simulink model "test_final_sift"  (R2015a)
settings: Solver=ode45  StartTime=0.0  StopTime=10.0  RelTol=1e-3
InitFcn:
  | %% DSPBuilder Start
  | alt_dspbuilder_update_model(bdroot)
  | %% DSPBuilder End
libraries: allblocks_alteradspbuilder2 x2309
(part 13 of 27)

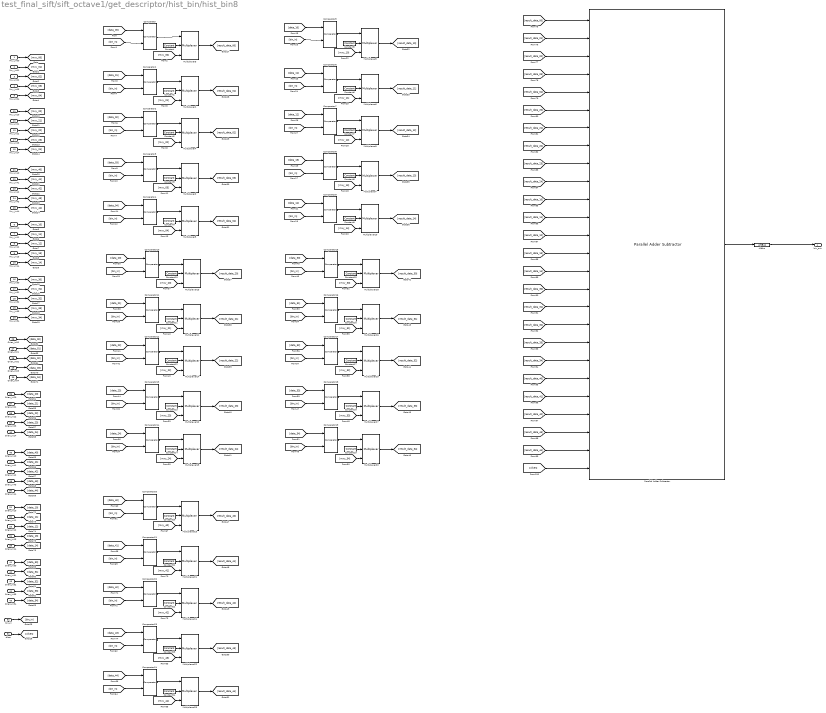
== system test_final_sift/sift_octave1/get_descriptor/hist_bin/hist_bin8 ==
  Mxy_In00 : Inport
  Mxy_In01 : Inport  Port=2
  Mxy_In02 : Inport  Port=3
  Mxy_In03 : Inport  Port=4
  Mxy_In04 : Inport  Port=5
  Mxy_In10 : Inport  Port=6
  Mxy_In11 : Inport  Port=7
  Mxy_In12 : Inport  Port=8
  Mxy_In13 : Inport  Port=9
  Mxy_In14 : Inport  Port=10
  Mxy_In20 : Inport  Port=11
  Mxy_In21 : Inport  Port=12
  Mxy_In22 : Inport  Port=13
  Mxy_In23 : Inport  Port=14
  Mxy_In24 : Inport  Port=15
  Mxy_In30 : Inport  Port=16
  Mxy_In31 : Inport  Port=17
  Mxy_In32 : Inport  Port=18
  Mxy_In33 : Inport  Port=19
  Mxy_In34 : Inport  Port=20
  Mxy_In40 : Inport  Port=21
  Mxy_In41 : Inport  Port=22
  Mxy_In42 : Inport  Port=23
  Mxy_In43 : Inport  Port=24
  Mxy_In44 : Inport  Port=25
  Orien_In00 : Inport  Port=26
  Orien_In01 : Inport  Port=27
  Orien_In02 : Inport  Port=28
  Orien_In03 : Inport  Port=29
  Orien_In04 : Inport  Port=30
  Orien_In10 : Inport  Port=31
  Orien_In11 : Inport  Port=32
  Orien_In12 : Inport  Port=33
  Orien_In13 : Inport  Port=34
  Orien_In14 : Inport  Port=35
  Orien_In20 : Inport  Port=36
  Orien_In21 : Inport  Port=37
  Orien_In22 : Inport  Port=38
  Orien_In23 : Inport  Port=39
  Orien_In24 : Inport  Port=40
  Orien_In30 : Inport  Port=41
  Orien_In31 : Inport  Port=42
  Orien_In32 : Inport  Port=43
  Orien_In33 : Inport  Port=44
  Orien_In34 : Inport  Port=45
  Orien_In40 : Inport  Port=46
  Orien_In41 : Inport  Port=47
  Orien_In42 : Inport  Port=48
  Orien_In43 : Inport  Port=49
  Orien_In44 : Inport  Port=50
  clken : Inport  Port=51
  bin_in : Inport  Port=52
  AltBus : allblocks_alteradspbuilder2/AltBus  BusType=Unsigned Integer  bwl=16  bwr=0  saturate=off  floatingPointInput=on  floatingPointOutput=on  logOutputs=off  logFile=C:\Users\ASUS\Desktop\sift_fpga\Octave_2\tb_test_final_sift\test%5Ffinal%5Fsift_sift%5Foctave1_get%5Fdescriptor_hist%5Fbin_hist%5Fbin8_AltBus.fixedpointlog
  Comparator : allblocks_alteradspbuilder2/Comparator  direction=a == b  pipeline_display=0  allowFloatingPointOverride=on  logOutputs=off  logFile=C:\Users\ASUS\Desktop\sift_fpga\Octave_2\tb_test_final_sift\test%5Ffinal%5Fsift_sift%5Foctave1_get%5Fdescriptor_hist%5Fbin_hist%5Fbin8_Comparator.fixedpointlog
  Comparator1 : allblocks_alteradspbuilder2/Comparator  direction=a == b  pipeline_display=0  allowFloatingPointOverride=on  logOutputs=off  logFile=C:\Users\ASUS\Desktop\sift_fpga\Octave_2\tb_test_final_sift\test%5Ffinal%5Fsift_sift%5Foctave1_get%5Fdescriptor_hist%5Fbin_hist%5Fbin8_Comparator1.fixedpointlog
  Comparator10 : allblocks_alteradspbuilder2/Comparator  direction=a == b  pipeline_display=0  allowFloatingPointOverride=on  logOutputs=off  logFile=C:\Users\ASUS\Desktop\sift_fpga\Octave_2\tb_test_final_sift\test%5Ffinal%5Fsift_sift%5Foctave1_get%5Fdescriptor_hist%5Fbin_hist%5Fbin8_Comparator10.fixedpointlog
  Comparator11 : allblocks_alteradspbuilder2/Comparator  direction=a == b  pipeline_display=0  allowFloatingPointOverride=on  logOutputs=off  logFile=C:\Users\ASUS\Desktop\sift_fpga\Octave_2\tb_test_final_sift\test%5Ffinal%5Fsift_sift%5Foctave1_get%5Fdescriptor_hist%5Fbin_hist%5Fbin8_Comparator11.fixedpointlog
  Comparator12 : allblocks_alteradspbuilder2/Comparator  direction=a == b  pipeline_display=0  allowFloatingPointOverride=on  logOutputs=off  logFile=C:\Users\ASUS\Desktop\sift_fpga\Octave_2\tb_test_final_sift\test%5Ffinal%5Fsift_sift%5Foctave1_get%5Fdescriptor_hist%5Fbin_hist%5Fbin8_Comparator12.fixedpointlog
  Comparator13 : allblocks_alteradspbuilder2/Comparator  direction=a == b  pipeline_display=0  allowFloatingPointOverride=on  logOutputs=off  logFile=C:\Users\ASUS\Desktop\sift_fpga\Octave_2\tb_test_final_sift\test%5Ffinal%5Fsift_sift%5Foctave1_get%5Fdescriptor_hist%5Fbin_hist%5Fbin8_Comparator13.fixedpointlog
  Comparator14 : allblocks_alteradspbuilder2/Comparator  direction=a == b  pipeline_display=0  allowFloatingPointOverride=on  logOutputs=off  logFile=C:\Users\ASUS\Desktop\sift_fpga\Octave_2\tb_test_final_sift\test%5Ffinal%5Fsift_sift%5Foctave1_get%5Fdescriptor_hist%5Fbin_hist%5Fbin8_Comparator14.fixedpointlog
  Comparator15 : allblocks_alteradspbuilder2/Comparator  direction=a == b  pipeline_display=0  allowFloatingPointOverride=on  logOutputs=off  logFile=C:\Users\ASUS\Desktop\sift_fpga\Octave_2\tb_test_final_sift\test%5Ffinal%5Fsift_sift%5Foctave1_get%5Fdescriptor_hist%5Fbin_hist%5Fbin8_Comparator15.fixedpointlog
  Comparator16 : allblocks_alteradspbuilder2/Comparator  direction=a == b  pipeline_display=0  allowFloatingPointOverride=on  logOutputs=off  logFile=C:\Users\ASUS\Desktop\sift_fpga\Octave_2\tb_test_final_sift\test%5Ffinal%5Fsift_sift%5Foctave1_get%5Fdescriptor_hist%5Fbin_hist%5Fbin8_Comparator16.fixedpointlog
  Comparator17 : allblocks_alteradspbuilder2/Comparator  direction=a == b  pipeline_display=0  allowFloatingPointOverride=on  logOutputs=off  logFile=C:\Users\ASUS\Desktop\sift_fpga\Octave_2\tb_test_final_sift\test%5Ffinal%5Fsift_sift%5Foctave1_get%5Fdescriptor_hist%5Fbin_hist%5Fbin8_Comparator17.fixedpointlog
  Comparator18 : allblocks_alteradspbuilder2/Comparator  direction=a == b  pipeline_display=0  allowFloatingPointOverride=on  logOutputs=off  logFile=C:\Users\ASUS\Desktop\sift_fpga\Octave_2\tb_test_final_sift\test%5Ffinal%5Fsift_sift%5Foctave1_get%5Fdescriptor_hist%5Fbin_hist%5Fbin8_Comparator18.fixedpointlog
  Comparator19 : allblocks_alteradspbuilder2/Comparator  direction=a == b  pipeline_display=0  allowFloatingPointOverride=on  logOutputs=off  logFile=C:\Users\ASUS\Desktop\sift_fpga\Octave_2\tb_test_final_sift\test%5Ffinal%5Fsift_sift%5Foctave1_get%5Fdescriptor_hist%5Fbin_hist%5Fbin8_Comparator19.fixedpointlog
  Comparator2 : allblocks_alteradspbuilder2/Comparator  direction=a == b  pipeline_display=0  allowFloatingPointOverride=on  logOutputs=off  logFile=C:\Users\ASUS\Desktop\sift_fpga\Octave_2\tb_test_final_sift\test%5Ffinal%5Fsift_sift%5Foctave1_get%5Fdescriptor_hist%5Fbin_hist%5Fbin8_Comparator2.fixedpointlog
  Comparator20 : allblocks_alteradspbuilder2/Comparator  direction=a == b  pipeline_display=0  allowFloatingPointOverride=on  logOutputs=off  logFile=C:\Users\ASUS\Desktop\sift_fpga\Octave_2\tb_test_final_sift\test%5Ffinal%5Fsift_sift%5Foctave1_get%5Fdescriptor_hist%5Fbin_hist%5Fbin8_Comparator20.fixedpointlog
  Comparator21 : allblocks_alteradspbuilder2/Comparator  direction=a == b  pipeline_display=0  allowFloatingPointOverride=on  logOutputs=off  logFile=C:\Users\ASUS\Desktop\sift_fpga\Octave_2\tb_test_final_sift\test%5Ffinal%5Fsift_sift%5Foctave1_get%5Fdescriptor_hist%5Fbin_hist%5Fbin8_Comparator21.fixedpointlog
  Comparator22 : allblocks_alteradspbuilder2/Comparator  direction=a == b  pipeline_display=0  allowFloatingPointOverride=on  logOutputs=off  logFile=C:\Users\ASUS\Desktop\sift_fpga\Octave_2\tb_test_final_sift\test%5Ffinal%5Fsift_sift%5Foctave1_get%5Fdescriptor_hist%5Fbin_hist%5Fbin8_Comparator22.fixedpointlog
  Comparator23 : allblocks_alteradspbuilder2/Comparator  direction=a == b  pipeline_display=0  allowFloatingPointOverride=on  logOutputs=off  logFile=C:\Users\ASUS\Desktop\sift_fpga\Octave_2\tb_test_final_sift\test%5Ffinal%5Fsift_sift%5Foctave1_get%5Fdescriptor_hist%5Fbin_hist%5Fbin8_Comparator23.fixedpointlog
  Comparator24 : allblocks_alteradspbuilder2/Comparator  direction=a == b  pipeline_display=0  allowFloatingPointOverride=on  logOutputs=off  logFile=C:\Users\ASUS\Desktop\sift_fpga\Octave_2\tb_test_final_sift\test%5Ffinal%5Fsift_sift%5Foctave1_get%5Fdescriptor_hist%5Fbin_hist%5Fbin8_Comparator24.fixedpointlog
  Comparator3 : allblocks_alteradspbuilder2/Comparator  direction=a == b  pipeline_display=0  allowFloatingPointOverride=on  logOutputs=off  logFile=C:\Users\ASUS\Desktop\sift_fpga\Octave_2\tb_test_final_sift\test%5Ffinal%5Fsift_sift%5Foctave1_get%5Fdescriptor_hist%5Fbin_hist%5Fbin8_Comparator3.fixedpointlog
  Comparator4 : allblocks_alteradspbuilder2/Comparator  direction=a == b  pipeline_display=0  allowFloatingPointOverride=on  logOutputs=off  logFile=C:\Users\ASUS\Desktop\sift_fpga\Octave_2\tb_test_final_sift\test%5Ffinal%5Fsift_sift%5Foctave1_get%5Fdescriptor_hist%5Fbin_hist%5Fbin8_Comparator4.fixedpointlog
  Comparator5 : allblocks_alteradspbuilder2/Comparator  direction=a == b  pipeline_display=0  allowFloatingPointOverride=on  logOutputs=off  logFile=C:\Users\ASUS\Desktop\sift_fpga\Octave_2\tb_test_final_sift\test%5Ffinal%5Fsift_sift%5Foctave1_get%5Fdescriptor_hist%5Fbin_hist%5Fbin8_Comparator5.fixedpointlog
  Comparator6 : allblocks_alteradspbuilder2/Comparator  direction=a == b  pipeline_display=0  allowFloatingPointOverride=on  logOutputs=off  logFile=C:\Users\ASUS\Desktop\sift_fpga\Octave_2\tb_test_final_sift\test%5Ffinal%5Fsift_sift%5Foctave1_get%5Fdescriptor_hist%5Fbin_hist%5Fbin8_Comparator6.fixedpointlog
  Comparator7 : allblocks_alteradspbuilder2/Comparator  direction=a == b  pipeline_display=0  allowFloatingPointOverride=on  logOutputs=off  logFile=C:\Users\ASUS\Desktop\sift_fpga\Octave_2\tb_test_final_sift\test%5Ffinal%5Fsift_sift%5Foctave1_get%5Fdescriptor_hist%5Fbin_hist%5Fbin8_Comparator7.fixedpointlog
  Comparator8 : allblocks_alteradspbuilder2/Comparator  direction=a == b  pipeline_display=0  allowFloatingPointOverride=on  logOutputs=off  logFile=C:\Users\ASUS\Desktop\sift_fpga\Octave_2\tb_test_final_sift\test%5Ffinal%5Fsift_sift%5Foctave1_get%5Fdescriptor_hist%5Fbin_hist%5Fbin8_Comparator8.fixedpointlog
  Comparator9 : allblocks_alteradspbuilder2/Comparator  direction=a == b  pipeline_display=0  allowFloatingPointOverride=on  logOutputs=off  logFile=C:\Users\ASUS\Desktop\sift_fpga\Octave_2\tb_test_final_sift\test%5Ffinal%5Fsift_sift%5Foctave1_get%5Fdescriptor_hist%5Fbin_hist%5Fbin8_Comparator9.fixedpointlog
  Constant : allblocks_alteradspbuilder2/Constant  mask_cst=0  BusType=Unsigned Integer  bwl=10  bwr=0  roundMode=Truncate  satMode=Wrap  SpecifyClock=off  allowFloatingPointOverride=on  logOutputs=off  logFile=C:\Users\ASUS\Desktop\sift_fpga\Octave_2\tb_test_final_sift\test%5Ffinal%5Fsift_sift%5Foctave1_get%5Fdescriptor_hist%5Fbin_hist%5Fbin8_Constant.fixedpointlog
  Constant1 : allblocks_alteradspbuilder2/Constant  mask_cst=0  BusType=Unsigned Integer  bwl=10  bwr=0  roundMode=Truncate  satMode=Wrap  SpecifyClock=off  allowFloatingPointOverride=on  logOutputs=off  logFile=C:\Users\ASUS\Desktop\sift_fpga\Octave_2\tb_test_final_sift\test%5Ffinal%5Fsift_sift%5Foctave1_get%5Fdescriptor_hist%5Fbin_hist%5Fbin8_Constant1.fixedpointlog
  Constant10 : allblocks_alteradspbuilder2/Constant  mask_cst=0  BusType=Unsigned Integer  bwl=10  bwr=0  roundMode=Truncate  satMode=Wrap  SpecifyClock=off  allowFloatingPointOverride=on  logOutputs=off  logFile=C:\Users\ASUS\Desktop\sift_fpga\Octave_2\tb_test_final_sift\test%5Ffinal%5Fsift_sift%5Foctave1_get%5Fdescriptor_hist%5Fbin_hist%5Fbin8_Constant10.fixedpointlog
  Constant11 : allblocks_alteradspbuilder2/Constant  mask_cst=0  BusType=Unsigned Integer  bwl=10  bwr=0  roundMode=Truncate  satMode=Wrap  SpecifyClock=off  allowFloatingPointOverride=on  logOutputs=off  logFile=C:\Users\ASUS\Desktop\sift_fpga\Octave_2\tb_test_final_sift\test%5Ffinal%5Fsift_sift%5Foctave1_get%5Fdescriptor_hist%5Fbin_hist%5Fbin8_Constant11.fixedpointlog
  Constant12 : allblocks_alteradspbuilder2/Constant  mask_cst=0  BusType=Unsigned Integer  bwl=10  bwr=0  roundMode=Truncate  satMode=Wrap  SpecifyClock=off  allowFloatingPointOverride=on  logOutputs=off  logFile=C:\Users\ASUS\Desktop\sift_fpga\Octave_2\tb_test_final_sift\test%5Ffinal%5Fsift_sift%5Foctave1_get%5Fdescriptor_hist%5Fbin_hist%5Fbin8_Constant12.fixedpointlog
  Constant13 : allblocks_alteradspbuilder2/Constant  mask_cst=0  BusType=Unsigned Integer  bwl=10  bwr=0  roundMode=Truncate  satMode=Wrap  SpecifyClock=off  allowFloatingPointOverride=on  logOutputs=off  logFile=C:\Users\ASUS\Desktop\sift_fpga\Octave_2\tb_test_final_sift\test%5Ffinal%5Fsift_sift%5Foctave1_get%5Fdescriptor_hist%5Fbin_hist%5Fbin8_Constant13.fixedpointlog
  Constant14 : allblocks_alteradspbuilder2/Constant  mask_cst=0  BusType=Unsigned Integer  bwl=10  bwr=0  roundMode=Truncate  satMode=Wrap  SpecifyClock=off  allowFloatingPointOverride=on  logOutputs=off  logFile=C:\Users\ASUS\Desktop\sift_fpga\Octave_2\tb_test_final_sift\test%5Ffinal%5Fsift_sift%5Foctave1_get%5Fdescriptor_hist%5Fbin_hist%5Fbin8_Constant14.fixedpointlog
  Constant15 : allblocks_alteradspbuilder2/Constant  mask_cst=0  BusType=Unsigned Integer  bwl=10  bwr=0  roundMode=Truncate  satMode=Wrap  SpecifyClock=off  allowFloatingPointOverride=on  logOutputs=off  logFile=C:\Users\ASUS\Desktop\sift_fpga\Octave_2\tb_test_final_sift\test%5Ffinal%5Fsift_sift%5Foctave1_get%5Fdescriptor_hist%5Fbin_hist%5Fbin8_Constant15.fixedpointlog
  Constant16 : allblocks_alteradspbuilder2/Constant  mask_cst=0  BusType=Unsigned Integer  bwl=10  bwr=0  roundMode=Truncate  satMode=Wrap  SpecifyClock=off  allowFloatingPointOverride=on  logOutputs=off  logFile=C:\Users\ASUS\Desktop\sift_fpga\Octave_2\tb_test_final_sift\test%5Ffinal%5Fsift_sift%5Foctave1_get%5Fdescriptor_hist%5Fbin_hist%5Fbin8_Constant16.fixedpointlog
  Constant17 : allblocks_alteradspbuilder2/Constant  mask_cst=0  BusType=Unsigned Integer  bwl=10  bwr=0  roundMode=Truncate  satMode=Wrap  SpecifyClock=off  allowFloatingPointOverride=on  logOutputs=off  logFile=C:\Users\ASUS\Desktop\sift_fpga\Octave_2\tb_test_final_sift\test%5Ffinal%5Fsift_sift%5Foctave1_get%5Fdescriptor_hist%5Fbin_hist%5Fbin8_Constant17.fixedpointlog
  Constant18 : allblocks_alteradspbuilder2/Constant  mask_cst=0  BusType=Unsigned Integer  bwl=10  bwr=0  roundMode=Truncate  satMode=Wrap  SpecifyClock=off  allowFloatingPointOverride=on  logOutputs=off  logFile=C:\Users\ASUS\Desktop\sift_fpga\Octave_2\tb_test_final_sift\test%5Ffinal%5Fsift_sift%5Foctave1_get%5Fdescriptor_hist%5Fbin_hist%5Fbin8_Constant18.fixedpointlog
  Constant19 : allblocks_alteradspbuilder2/Constant  mask_cst=0  BusType=Unsigned Integer  bwl=10  bwr=0  roundMode=Truncate  satMode=Wrap  SpecifyClock=off  allowFloatingPointOverride=on  logOutputs=off  logFile=C:\Users\ASUS\Desktop\sift_fpga\Octave_2\tb_test_final_sift\test%5Ffinal%5Fsift_sift%5Foctave1_get%5Fdescriptor_hist%5Fbin_hist%5Fbin8_Constant19.fixedpointlog
  Constant2 : allblocks_alteradspbuilder2/Constant  mask_cst=0  BusType=Unsigned Integer  bwl=10  bwr=0  roundMode=Truncate  satMode=Wrap  SpecifyClock=off  allowFloatingPointOverride=on  logOutputs=off  logFile=C:\Users\ASUS\Desktop\sift_fpga\Octave_2\tb_test_final_sift\test%5Ffinal%5Fsift_sift%5Foctave1_get%5Fdescriptor_hist%5Fbin_hist%5Fbin8_Constant2.fixedpointlog
  Constant20 : allblocks_alteradspbuilder2/Constant  mask_cst=0  BusType=Unsigned Integer  bwl=10  bwr=0  roundMode=Truncate  satMode=Wrap  SpecifyClock=off  allowFloatingPointOverride=on  logOutputs=off  logFile=C:\Users\ASUS\Desktop\sift_fpga\Octave_2\tb_test_final_sift\test%5Ffinal%5Fsift_sift%5Foctave1_get%5Fdescriptor_hist%5Fbin_hist%5Fbin8_Constant20.fixedpointlog
  Constant21 : allblocks_alteradspbuilder2/Constant  mask_cst=0  BusType=Unsigned Integer  bwl=10  bwr=0  roundMode=Truncate  satMode=Wrap  SpecifyClock=off  allowFloatingPointOverride=on  logOutputs=off  logFile=C:\Users\ASUS\Desktop\sift_fpga\Octave_2\tb_test_final_sift\test%5Ffinal%5Fsift_sift%5Foctave1_get%5Fdescriptor_hist%5Fbin_hist%5Fbin8_Constant21.fixedpointlog
  Constant22 : allblocks_alteradspbuilder2/Constant  mask_cst=0  BusType=Unsigned Integer  bwl=10  bwr=0  roundMode=Truncate  satMode=Wrap  SpecifyClock=off  allowFloatingPointOverride=on  logOutputs=off  logFile=C:\Users\ASUS\Desktop\sift_fpga\Octave_2\tb_test_final_sift\test%5Ffinal%5Fsift_sift%5Foctave1_get%5Fdescriptor_hist%5Fbin_hist%5Fbin8_Constant22.fixedpointlog
  Constant23 : allblocks_alteradspbuilder2/Constant  mask_cst=0  BusType=Unsigned Integer  bwl=10  bwr=0  roundMode=Truncate  satMode=Wrap  SpecifyClock=off  allowFloatingPointOverride=on  logOutputs=off  logFile=C:\Users\ASUS\Desktop\sift_fpga\Octave_2\tb_test_final_sift\test%5Ffinal%5Fsift_sift%5Foctave1_get%5Fdescriptor_hist%5Fbin_hist%5Fbin8_Constant23.fixedpointlog
  Constant24 : allblocks_alteradspbuilder2/Constant  mask_cst=0  BusType=Unsigned Integer  bwl=10  bwr=0  roundMode=Truncate  satMode=Wrap  SpecifyClock=off  allowFloatingPointOverride=on  logOutputs=off  logFile=C:\Users\ASUS\Desktop\sift_fpga\Octave_2\tb_test_final_sift\test%5Ffinal%5Fsift_sift%5Foctave1_get%5Fdescriptor_hist%5Fbin_hist%5Fbin8_Constant24.fixedpointlog
  Constant3 : allblocks_alteradspbuilder2/Constant  mask_cst=0  BusType=Unsigned Integer  bwl=10  bwr=0  roundMode=Truncate  satMode=Wrap  SpecifyClock=off  allowFloatingPointOverride=on  logOutputs=off  logFile=C:\Users\ASUS\Desktop\sift_fpga\Octave_2\tb_test_final_sift\test%5Ffinal%5Fsift_sift%5Foctave1_get%5Fdescriptor_hist%5Fbin_hist%5Fbin8_Constant3.fixedpointlog
  Constant4 : allblocks_alteradspbuilder2/Constant  mask_cst=0  BusType=Unsigned Integer  bwl=10  bwr=0  roundMode=Truncate  satMode=Wrap  SpecifyClock=off  allowFloatingPointOverride=on  logOutputs=off  logFile=C:\Users\ASUS\Desktop\sift_fpga\Octave_2\tb_test_final_sift\test%5Ffinal%5Fsift_sift%5Foctave1_get%5Fdescriptor_hist%5Fbin_hist%5Fbin8_Constant4.fixedpointlog
  Constant5 : allblocks_alteradspbuilder2/Constant  mask_cst=0  BusType=Unsigned Integer  bwl=10  bwr=0  roundMode=Truncate  satMode=Wrap  SpecifyClock=off  allowFloatingPointOverride=on  logOutputs=off  logFile=C:\Users\ASUS\Desktop\sift_fpga\Octave_2\tb_test_final_sift\test%5Ffinal%5Fsift_sift%5Foctave1_get%5Fdescriptor_hist%5Fbin_hist%5Fbin8_Constant5.fixedpointlog
  Constant6 : allblocks_alteradspbuilder2/Constant  mask_cst=0  BusType=Unsigned Integer  bwl=10  bwr=0  roundMode=Truncate  satMode=Wrap  SpecifyClock=off  allowFloatingPointOverride=on  logOutputs=off  logFile=C:\Users\ASUS\Desktop\sift_fpga\Octave_2\tb_test_final_sift\test%5Ffinal%5Fsift_sift%5Foctave1_get%5Fdescriptor_hist%5Fbin_hist%5Fbin8_Constant6.fixedpointlog
  Constant7 : allblocks_alteradspbuilder2/Constant  mask_cst=0  BusType=Unsigned Integer  bwl=10  bwr=0  roundMode=Truncate  satMode=Wrap  SpecifyClock=off  allowFloatingPointOverride=on  logOutputs=off  logFile=C:\Users\ASUS\Desktop\sift_fpga\Octave_2\tb_test_final_sift\test%5Ffinal%5Fsift_sift%5Foctave1_get%5Fdescriptor_hist%5Fbin_hist%5Fbin8_Constant7.fixedpointlog
  Constant8 : allblocks_alteradspbuilder2/Constant  mask_cst=0  BusType=Unsigned Integer  bwl=10  bwr=0  roundMode=Truncate  satMode=Wrap  SpecifyClock=off  allowFloatingPointOverride=on  logOutputs=off  logFile=C:\Users\ASUS\Desktop\sift_fpga\Octave_2\tb_test_final_sift\test%5Ffinal%5Fsift_sift%5Foctave1_get%5Fdescriptor_hist%5Fbin_hist%5Fbin8_Constant8.fixedpointlog
  Constant9 : allblocks_alteradspbuilder2/Constant  mask_cst=0  BusType=Unsigned Integer  bwl=10  bwr=0  roundMode=Truncate  satMode=Wrap  SpecifyClock=off  allowFloatingPointOverride=on  logOutputs=off  logFile=C:\Users\ASUS\Desktop\sift_fpga\Octave_2\tb_test_final_sift\test%5Ffinal%5Fsift_sift%5Foctave1_get%5Fdescriptor_hist%5Fbin_hist%5Fbin8_Constant9.fixedpointlog
  Multiplexer1 : allblocks_alteradspbuilder2/Multiplexer  numInputs=2  pipeline=0  oneHot=off  pipeline_display=0  use_ena=off  use_aclr=off  allowFloatingPointOverride=on  logOutputs=off  logFile=C:\Users\ASUS\Desktop\sift_fpga\Octave_2\tb_test_final_sift\test%5Ffinal%5Fsift_sift%5Foctave1_get%5Fdescriptor_hist%5Fbin_hist%5Fbin8_Multiplexer1.fixedpointlog
  Multiplexer10 : allblocks_alteradspbuilder2/Multiplexer  numInputs=2  pipeline=0  oneHot=off  pipeline_display=0  use_ena=off  use_aclr=off  allowFloatingPointOverride=on  logOutputs=off  logFile=C:\Users\ASUS\Desktop\sift_fpga\Octave_2\tb_test_final_sift\test%5Ffinal%5Fsift_sift%5Foctave1_get%5Fdescriptor_hist%5Fbin_hist%5Fbin8_Multiplexer10.fixedpointlog
  Multiplexer11 : allblocks_alteradspbuilder2/Multiplexer  numInputs=2  pipeline=0  oneHot=off  pipeline_display=0  use_ena=off  use_aclr=off  allowFloatingPointOverride=on  logOutputs=off  logFile=C:\Users\ASUS\Desktop\sift_fpga\Octave_2\tb_test_final_sift\test%5Ffinal%5Fsift_sift%5Foctave1_get%5Fdescriptor_hist%5Fbin_hist%5Fbin8_Multiplexer11.fixedpointlog
  Multiplexer12 : allblocks_alteradspbuilder2/Multiplexer  numInputs=2  pipeline=0  oneHot=off  pipeline_display=0  use_ena=off  use_aclr=off  allowFloatingPointOverride=on  logOutputs=off  logFile=C:\Users\ASUS\Desktop\sift_fpga\Octave_2\tb_test_final_sift\test%5Ffinal%5Fsift_sift%5Foctave1_get%5Fdescriptor_hist%5Fbin_hist%5Fbin8_Multiplexer12.fixedpointlog
  Multiplexer13 : allblocks_alteradspbuilder2/Multiplexer  numInputs=2  pipeline=0  oneHot=off  pipeline_display=0  use_ena=off  use_aclr=off  allowFloatingPointOverride=on  logOutputs=off  logFile=C:\Users\ASUS\Desktop\sift_fpga\Octave_2\tb_test_final_sift\test%5Ffinal%5Fsift_sift%5Foctave1_get%5Fdescriptor_hist%5Fbin_hist%5Fbin8_Multiplexer13.fixedpointlog
  Multiplexer14 : allblocks_alteradspbuilder2/Multiplexer  numInputs=2  pipeline=0  oneHot=off  pipeline_display=0  use_ena=off  use_aclr=off  allowFloatingPointOverride=on  logOutputs=off  logFile=C:\Users\ASUS\Desktop\sift_fpga\Octave_2\tb_test_final_sift\test%5Ffinal%5Fsift_sift%5Foctave1_get%5Fdescriptor_hist%5Fbin_hist%5Fbin8_Multiplexer14.fixedpointlog
  Multiplexer15 : allblocks_alteradspbuilder2/Multiplexer  numInputs=2  pipeline=0  oneHot=off  pipeline_display=0  use_ena=off  use_aclr=off  allowFloatingPointOverride=on  logOutputs=off  logFile=C:\Users\ASUS\Desktop\sift_fpga\Octave_2\tb_test_final_sift\test%5Ffinal%5Fsift_sift%5Foctave1_get%5Fdescriptor_hist%5Fbin_hist%5Fbin8_Multiplexer15.fixedpointlog
  Multiplexer16 : allblocks_alteradspbuilder2/Multiplexer  numInputs=2  pipeline=0  oneHot=off  pipeline_display=0  use_ena=off  use_aclr=off  allowFloatingPointOverride=on  logOutputs=off  logFile=C:\Users\ASUS\Desktop\sift_fpga\Octave_2\tb_test_final_sift\test%5Ffinal%5Fsift_sift%5Foctave1_get%5Fdescriptor_hist%5Fbin_hist%5Fbin8_Multiplexer16.fixedpointlog
  Multiplexer17 : allblocks_alteradspbuilder2/Multiplexer  numInputs=2  pipeline=0  oneHot=off  pipeline_display=0  use_ena=off  use_aclr=off  allowFloatingPointOverride=on  logOutputs=off  logFile=C:\Users\ASUS\Desktop\sift_fpga\Octave_2\tb_test_final_sift\test%5Ffinal%5Fsift_sift%5Foctave1_get%5Fdescriptor_hist%5Fbin_hist%5Fbin8_Multiplexer17.fixedpointlog
  Multiplexer18 : allblocks_alteradspbuilder2/Multiplexer  numInputs=2  pipeline=0  oneHot=off  pipeline_display=0  use_ena=off  use_aclr=off  allowFloatingPointOverride=on  logOutputs=off  logFile=C:\Users\ASUS\Desktop\sift_fpga\Octave_2\tb_test_final_sift\test%5Ffinal%5Fsift_sift%5Foctave1_get%5Fdescriptor_hist%5Fbin_hist%5Fbin8_Multiplexer18.fixedpointlog
  Multiplexer19 : allblocks_alteradspbuilder2/Multiplexer  numInputs=2  pipeline=0  oneHot=off  pipeline_display=0  use_ena=off  use_aclr=off  allowFloatingPointOverride=on  logOutputs=off  logFile=C:\Users\ASUS\Desktop\sift_fpga\Octave_2\tb_test_final_sift\test%5Ffinal%5Fsift_sift%5Foctave1_get%5Fdescriptor_hist%5Fbin_hist%5Fbin8_Multiplexer19.fixedpointlog
  Multiplexer2 : allblocks_alteradspbuilder2/Multiplexer  numInputs=2  pipeline=0  oneHot=off  pipeline_display=0  use_ena=off  use_aclr=off  allowFloatingPointOverride=on  logOutputs=off  logFile=C:\Users\ASUS\Desktop\sift_fpga\Octave_2\tb_test_final_sift\test%5Ffinal%5Fsift_sift%5Foctave1_get%5Fdescriptor_hist%5Fbin_hist%5Fbin8_Multiplexer2.fixedpointlog
  Multiplexer20 : allblocks_alteradspbuilder2/Multiplexer  numInputs=2  pipeline=0  oneHot=off  pipeline_display=0  use_ena=off  use_aclr=off  allowFloatingPointOverride=on  logOutputs=off  logFile=C:\Users\ASUS\Desktop\sift_fpga\Octave_2\tb_test_final_sift\test%5Ffinal%5Fsift_sift%5Foctave1_get%5Fdescriptor_hist%5Fbin_hist%5Fbin8_Multiplexer20.fixedpointlog
  Multiplexer21 : allblocks_alteradspbuilder2/Multiplexer  numInputs=2  pipeline=0  oneHot=off  pipeline_display=0  use_ena=off  use_aclr=off  allowFloatingPointOverride=on  logOutputs=off  logFile=C:\Users\ASUS\Desktop\sift_fpga\Octave_2\tb_test_final_sift\test%5Ffinal%5Fsift_sift%5Foctave1_get%5Fdescriptor_hist%5Fbin_hist%5Fbin8_Multiplexer21.fixedpointlog
  Multiplexer22 : allblocks_alteradspbuilder2/Multiplexer  numInputs=2  pipeline=0  oneHot=off  pipeline_display=0  use_ena=off  use_aclr=off  allowFloatingPointOverride=on  logOutputs=off  logFile=C:\Users\ASUS\Desktop\sift_fpga\Octave_2\tb_test_final_sift\test%5Ffinal%5Fsift_sift%5Foctave1_get%5Fdescriptor_hist%5Fbin_hist%5Fbin8_Multiplexer22.fixedpointlog
  Multiplexer23 : allblocks_alteradspbuilder2/Multiplexer  numInputs=2  pipeline=0  oneHot=off  pipeline_display=0  use_ena=off  use_aclr=off  allowFloatingPointOverride=on  logOutputs=off  logFile=C:\Users\ASUS\Desktop\sift_fpga\Octave_2\tb_test_final_sift\test%5Ffinal%5Fsift_sift%5Foctave1_get%5Fdescriptor_hist%5Fbin_hist%5Fbin8_Multiplexer23.fixedpointlog
  Multiplexer24 : allblocks_alteradspbuilder2/Multiplexer  numInputs=2  pipeline=0  oneHot=off  pipeline_display=0  use_ena=off  use_aclr=off  allowFloatingPointOverride=on  logOutputs=off  logFile=C:\Users\ASUS\Desktop\sift_fpga\Octave_2\tb_test_final_sift\test%5Ffinal%5Fsift_sift%5Foctave1_get%5Fdescriptor_hist%5Fbin_hist%5Fbin8_Multiplexer24.fixedpointlog
  Multiplexer25 : allblocks_alteradspbuilder2/Multiplexer  numInputs=2  pipeline=0  oneHot=off  pipeline_display=0  use_ena=off  use_aclr=off  allowFloatingPointOverride=on  logOutputs=off  logFile=C:\Users\ASUS\Desktop\sift_fpga\Octave_2\tb_test_final_sift\test%5Ffinal%5Fsift_sift%5Foctave1_get%5Fdescriptor_hist%5Fbin_hist%5Fbin8_Multiplexer25.fixedpointlog
  Multiplexer3 : allblocks_alteradspbuilder2/Multiplexer  numInputs=2  pipeline=0  oneHot=off  pipeline_display=0  use_ena=off  use_aclr=off  allowFloatingPointOverride=on  logOutputs=off  logFile=C:\Users\ASUS\Desktop\sift_fpga\Octave_2\tb_test_final_sift\test%5Ffinal%5Fsift_sift%5Foctave1_get%5Fdescriptor_hist%5Fbin_hist%5Fbin8_Multiplexer3.fixedpointlog
  Multiplexer4 : allblocks_alteradspbuilder2/Multiplexer  numInputs=2  pipeline=0  oneHot=off  pipeline_display=0  use_ena=off  use_aclr=off  allowFloatingPointOverride=on  logOutputs=off  logFile=C:\Users\ASUS\Desktop\sift_fpga\Octave_2\tb_test_final_sift\test%5Ffinal%5Fsift_sift%5Foctave1_get%5Fdescriptor_hist%5Fbin_hist%5Fbin8_Multiplexer4.fixedpointlog
  Multiplexer5 : allblocks_alteradspbuilder2/Multiplexer  numInputs=2  pipeline=0  oneHot=off  pipeline_display=0  use_ena=off  use_aclr=off  allowFloatingPointOverride=on  logOutputs=off  logFile=C:\Users\ASUS\Desktop\sift_fpga\Octave_2\tb_test_final_sift\test%5Ffinal%5Fsift_sift%5Foctave1_get%5Fdescriptor_hist%5Fbin_hist%5Fbin8_Multiplexer5.fixedpointlog
  Multiplexer6 : allblocks_alteradspbuilder2/Multiplexer  numInputs=2  pipeline=0  oneHot=off  pipeline_display=0  use_ena=off  use_aclr=off  allowFloatingPointOverride=on  logOutputs=off  logFile=C:\Users\ASUS\Desktop\sift_fpga\Octave_2\tb_test_final_sift\test%5Ffinal%5Fsift_sift%5Foctave1_get%5Fdescriptor_hist%5Fbin_hist%5Fbin8_Multiplexer6.fixedpointlog
  Multiplexer7 : allblocks_alteradspbuilder2/Multiplexer  numInputs=2  pipeline=0  oneHot=off  pipeline_display=0  use_ena=off  use_aclr=off  allowFloatingPointOverride=on  logOutputs=off  logFile=C:\Users\ASUS\Desktop\sift_fpga\Octave_2\tb_test_final_sift\test%5Ffinal%5Fsift_sift%5Foctave1_get%5Fdescriptor_hist%5Fbin_hist%5Fbin8_Multiplexer7.fixedpointlog
  Multiplexer8 : allblocks_alteradspbuilder2/Multiplexer  numInputs=2  pipeline=0  oneHot=off  pipeline_display=0  use_ena=off  use_aclr=off  allowFloatingPointOverride=on  logOutputs=off  logFile=C:\Users\ASUS\Desktop\sift_fpga\Octave_2\tb_test_final_sift\test%5Ffinal%5Fsift_sift%5Foctave1_get%5Fdescriptor_hist%5Fbin_hist%5Fbin8_Multiplexer8.fixedpointlog
  Multiplexer9 : allblocks_alteradspbuilder2/Multiplexer  numInputs=2  pipeline=0  oneHot=off  pipeline_display=0  use_ena=off  use_aclr=off  allowFloatingPointOverride=on  logOutputs=off  logFile=C:\Users\ASUS\Desktop\sift_fpga\Octave_2\tb_test_final_sift\test%5Ffinal%5Fsift_sift%5Foctave1_get%5Fdescriptor_hist%5Fbin_hist%5Fbin8_Multiplexer9.fixedpointlog
  Parallel Adder Subtractor : allblocks_alteradspbuilder2/Parallel Adder Subtractor  number_of_inputs=25  direction=+  use_pipeline=on  pipeline_display=5  phase_selection=1  use_ena=on  use_aclr=off  allowFloatingPointOverride=on  logOutputs=off  logFile=C:\Users\ASUS\Desktop\sift_fpga\Octave_2\tb_test_final_sift\test%5Ffinal%5Fsift_sift%5Foctave1_get%5Fdescriptor_hist%5Fbin_hist%5Fbin8_Parallel+Adder+Subtractor.fixedpointlog
  bin_out : Outport
  wires:
  Mxy_In00/1 -> [mxy_00]
  Mxy_In21/1 -> [mxy_21]
  Mxy_In30/1 -> [mxy_30]
  Mxy_In04/1 -> [mxy_04]
  Mxy_In03/1 -> [mxy_03]
  Mxy_In14/1 -> [mxy_14]
  Mxy_In02/1 -> [mxy_02]
  Mxy_In13/1 -> [mxy_13]
  Mxy_In31/1 -> [mxy_31]
  Mxy_In20/1 -> [mxy_20]
  Mxy_In22/1 -> [mxy_22]
  Mxy_In24/1 -> [mxy_24]
  Mxy_In23/1 -> [mxy_23]
  Mxy_In01/1 -> [mxy_01]
  Mxy_In32/1 -> [mxy_32]
  Mxy_In34/1 -> [mxy_34]
  Mxy_In33/1 -> [mxy_33]
  Mxy_In40/1 -> [mxy_40]
  Mxy_In41/1 -> [mxy_41]
  Mxy_In42/1 -> [mxy_42]
  Mxy_In44/1 -> [mxy_44]
  Mxy_In12/1 -> [mxy_12]
  Mxy_In11/1 -> [mxy_11]
  Mxy_In10/1 -> [mxy_10]
  Mxy_In43/1 -> [mxy_43]
  [data_00] -> Comparator/1
  [bin_in] -> Comparator/2
  Comparator/1 -> Multiplexer3/1
  [mxy_00] -> Multiplexer3/3
  Constant/1 -> Multiplexer3/2
  Multiplexer3/1 -> [result_data_00]
  [data_01] -> Comparator1/1
  [bin_in] -> Comparator1/2
  Comparator1/1 -> Multiplexer1/1
  [mxy_01] -> Multiplexer1/3
  Constant1/1 -> Multiplexer1/2
  Multiplexer1/1 -> [result_data_01]
  [data_02] -> Comparator2/1
  [bin_in] -> Comparator2/2
  Comparator2/1 -> Multiplexer4/1
  [mxy_02] -> Multiplexer4/3
  Constant2/1 -> Multiplexer4/2
  Multiplexer4/1 -> [result_data_02]
  [data_03] -> Comparator3/1
  [bin_in] -> Comparator3/2
  Comparator3/1 -> Multiplexer2/1
  [mxy_03] -> Multiplexer2/3
  Constant3/1 -> Multiplexer2/2
  Multiplexer2/1 -> [result_data_03]
  [data_04] -> Comparator4/1
  [bin_in] -> Comparator4/2
  Comparator4/1 -> Multiplexer5/1
  [mxy_04] -> Multiplexer5/3
  Constant4/1 -> Multiplexer5/2
  Multiplexer5/1 -> [result_data_04]
  [data_10] -> Comparator5/1
  [bin_in] -> Comparator5/2
  Comparator5/1 -> Multiplexer8/1
  [mxy_10] -> Multiplexer8/3
  Constant5/1 -> Multiplexer8/2
  Multiplexer8/1 -> [result_data_10]
  [data_11] -> Comparator6/1
  [bin_in] -> Comparator6/2
  Comparator6/1 -> Multiplexer6/1
  [mxy_11] -> Multiplexer6/3
  Constant6/1 -> Multiplexer6/2
  Multiplexer6/1 -> [result_data_11]
  [data_12] -> Comparator7/1
  [bin_in] -> Comparator7/2
  Comparator7/1 -> Multiplexer9/1
  [mxy_12] -> Multiplexer9/3
  Constant7/1 -> Multiplexer9/2
  Multiplexer9/1 -> [result_data_12]
  [data_13] -> Comparator8/1
  [bin_in] -> Comparator8/2
  Comparator8/1 -> Multiplexer7/1
  [mxy_13] -> Multiplexer7/3
  Constant8/1 -> Multiplexer7/2
  Multiplexer7/1 -> [result_data_13]
  [data_14] -> Comparator9/1
  [bin_in] -> Comparator9/2
  Comparator9/1 -> Multiplexer10/1
  [mxy_14] -> Multiplexer10/3
  Constant9/1 -> Multiplexer10/2
  Multiplexer10/1 -> [result_data_14]
  [data_20] -> Comparator10/1
  [bin_in] -> Comparator10/2
  Comparator10/1 -> Multiplexer13/1
  [mxy_20] -> Multiplexer13/3
  Constant10/1 -> Multiplexer13/2
  Multiplexer13/1 -> [result_data_20]
  [data_21] -> Comparator11/1
  [bin_in] -> Comparator11/2
  Comparator11/1 -> Multiplexer11/1
  [mxy_21] -> Multiplexer11/3
  Constant11/1 -> Multiplexer11/2
  Multiplexer11/1 -> [result_data_21]
  [data_22] -> Comparator12/1
  [bin_in] -> Comparator12/2
  Comparator12/1 -> Multiplexer14/1
  [mxy_22] -> Multiplexer14/3
  Constant12/1 -> Multiplexer14/2
  Multiplexer14/1 -> [result_data_22]
  [data_23] -> Comparator13/1
  [bin_in] -> Comparator13/2
  Comparator13/1 -> Multiplexer12/1
  [mxy_23] -> Multiplexer12/3
  Constant13/1 -> Multiplexer12/2
  Multiplexer12/1 -> [result_data_23]
  [data_24] -> Comparator14/1
  [bin_in] -> Comparator14/2
  Comparator14/1 -> Multiplexer15/1
  [mxy_24] -> Multiplexer15/3
  Constant14/1 -> Multiplexer15/2
  Multiplexer15/1 -> [result_data_24]
  [data_30] -> Comparator15/1
  [bin_in] -> Comparator15/2
  Comparator15/1 -> Multiplexer18/1
  [mxy_30] -> Multiplexer18/3
  Constant15/1 -> Multiplexer18/2
  Multiplexer18/1 -> [result_data_30]
  [data_31] -> Comparator16/1
  [bin_in] -> Comparator16/2
  Comparator16/1 -> Multiplexer16/1
  [mxy_31] -> Multiplexer16/3
  Constant16/1 -> Multiplexer16/2
  Multiplexer16/1 -> [result_data_31]
  [data_32] -> Comparator17/1
  [bin_in] -> Comparator17/2
  Comparator17/1 -> Multiplexer19/1
  [mxy_32] -> Multiplexer19/3
  Constant17/1 -> Multiplexer19/2
  Multiplexer19/1 -> [result_data_32]
  [data_33] -> Comparator18/1
  [bin_in] -> Comparator18/2
  Comparator18/1 -> Multiplexer17/1
  [mxy_33] -> Multiplexer17/3
  Constant18/1 -> Multiplexer17/2
  Multiplexer17/1 -> [result_data_33]
  [data_34] -> Comparator19/1
  [bin_in] -> Comparator19/2
  Comparator19/1 -> Multiplexer20/1
  [mxy_34] -> Multiplexer20/3
  Constant19/1 -> Multiplexer20/2
  Multiplexer20/1 -> [result_data_34]
  [data_40] -> Comparator20/1
  [bin_in] -> Comparator20/2
  Comparator20/1 -> Multiplexer23/1
  [mxy_40] -> Multiplexer23/3
  Constant20/1 -> Multiplexer23/2
  Multiplexer23/1 -> [result_data_40]
  [data_41] -> Comparator21/1
  [bin_in] -> Comparator21/2
  Comparator21/1 -> Multiplexer21/1
  [mxy_41] -> Multiplexer21/3
  Constant21/1 -> Multiplexer21/2
  Multiplexer21/1 -> [result_data_41]
  [data_42] -> Comparator22/1
  [bin_in] -> Comparator22/2
  Comparator22/1 -> Multiplexer24/1
  [mxy_42] -> Multiplexer24/3
  Constant22/1 -> Multiplexer24/2
  Multiplexer24/1 -> [result_data_42]
  [data_43] -> Comparator23/1
  [bin_in] -> Comparator23/2
  Comparator23/1 -> Multiplexer22/1
  [mxy_43] -> Multiplexer22/3
  Constant23/1 -> Multiplexer22/2
  Multiplexer22/1 -> [result_data_43]
  [data_44] -> Comparator24/1
  [bin_in] -> Comparator24/2
  Comparator24/1 -> Multiplexer25/1
  [mxy_44] -> Multiplexer25/3
  Constant24/1 -> Multiplexer25/2
  Multiplexer25/1 -> [result_data_44]
  Orien_In00/1 -> [data_00]
  Orien_In21/1 -> [data_21]
  Orien_In30/1 -> [data_30]
  Orien_In04/1 -> [data_04]
  Orien_In03/1 -> [data_03]
  Orien_In14/1 -> [data_14]
  Orien_In02/1 -> [data_02]
  Orien_In13/1 -> [data_13]
  Orien_In31/1 -> [data_31]
  Orien_In20/1 -> [data_20]
  Orien_In22/1 -> [data_22]
  Orien_In24/1 -> [data_24]
  Orien_In23/1 -> [data_23]
  Orien_In01/1 -> [data_01]
  Orien_In32/1 -> [data_32]
  Orien_In34/1 -> [data_34]
  Orien_In33/1 -> [data_33]
  Orien_In40/1 -> [data_40]
  Orien_In41/1 -> [data_41]
  Orien_In42/1 -> [data_42]
  Orien_In44/1 -> [data_44]
  Orien_In12/1 -> [data_12]
  Orien_In11/1 -> [data_11]
  Orien_In10/1 -> [data_10]
  Orien_In43/1 -> [data_43]
  clken/1 -> [clken]
  bin_in/1 -> [bin_in]
  [result_data_00] -> Parallel Adder Subtractor/1
  [result_data_01] -> Parallel Adder Subtractor/2
  [result_data_02] -> Parallel Adder Subtractor/3
  [result_data_03] -> Parallel Adder Subtractor/4
  [result_data_04] -> Parallel Adder Subtractor/5
  [result_data_20] -> Parallel Adder Subtractor/6
  [result_data_21] -> Parallel Adder Subtractor/7
  [result_data_22] -> Parallel Adder Subtractor/8
  [result_data_23] -> Parallel Adder Subtractor/9
  [result_data_24] -> Parallel Adder Subtractor/10
  [result_data_10] -> Parallel Adder Subtractor/11
  [result_data_11] -> Parallel Adder Subtractor/12
  [result_data_12] -> Parallel Adder Subtractor/13
  [result_data_13] -> Parallel Adder Subtractor/14
  [result_data_14] -> Parallel Adder Subtractor/15
  [result_data_30] -> Parallel Adder Subtractor/16
  [result_data_31] -> Parallel Adder Subtractor/17
  [result_data_32] -> Parallel Adder Subtractor/18
  [result_data_33] -> Parallel Adder Subtractor/19
  [result_data_34] -> Parallel Adder Subtractor/20
  [result_data_40] -> Parallel Adder Subtractor/21
  [result_data_41] -> Parallel Adder Subtractor/22
  [result_data_42] -> Parallel Adder Subtractor/23
  [result_data_43] -> Parallel Adder Subtractor/24
  [result_data_44] -> Parallel Adder Subtractor/25
  [clken] -> Parallel Adder Subtractor/26
  Parallel Adder Subtractor/1 -> AltBus/1
  AltBus/1 -> bin_out/1

== system test_final_sift/sift_octave1/get_descriptor/scale_space/Gaussian_scale1 ==
  pixel_in : Inport
  valid_in : Inport  Port=2
  Mul : Subsystem
  Round : allblocks_alteradspbuilder2/Round  BusType=Signed Fractional  bwl=9  bwr=16  bitsToRemove=0  roundMode=TRUNCATE_LOW  userRoundMode=Truncate  pipeline=off  pipeline_display=0  use_ena=off  use_aclr=off
  line_buff : Subsystem
  pixel_out : Outport
  wires:
  line_buff/20(Out34) -> Mul/20(In34)
  line_buff/7(Out11) -> Mul/7(In11)
  line_buff/22(Out41) -> Mul/22(In41)
  line_buff/21(Out40) -> Mul/21(In40)
  line_buff/23(Out42) -> Mul/23(In42)
  line_buff/24(Out43) -> Mul/24(In43)
  line_buff/6(Out10) -> Mul/6(In10)
  line_buff/19(Out33) -> Mul/19(In33)
  line_buff/25(Out44) -> Mul/25(In44)
  line_buff/11(Out20) -> Mul/11(In20)
  line_buff/1(Out00) -> Mul/1(In00)
  line_buff/5(Out04) -> Mul/5(In04)
  pixel_in/1 -> line_buff/1(dataIn)
  line_buff/13(Out22) -> Mul/13(In22)
  line_buff/16(Out30) -> Mul/16(In30)
  line_buff/18(Out32) -> Mul/18(In32)
  Mul/1(pixel) -> Round/1
  line_buff/10(Out14) -> Mul/10(In14)
  valid_in/1 -> Mul/26(clken), line_buff/2(clken)
  line_buff/12(Out21) -> Mul/12(In21)
  line_buff/14(Out23) -> Mul/14(In23)
  line_buff/2(Out01) -> Mul/2(In01)
  line_buff/4(Out03) -> Mul/4(In03)
  line_buff/9(Out13) -> Mul/9(In13)
  line_buff/15(Out24) -> Mul/15(In24)
  line_buff/17(Out31) -> Mul/17(In31)
  line_buff/3(Out02) -> Mul/3(In02)
  line_buff/8(Out12) -> Mul/8(In12)
  Round/1 -> pixel_out/1

== system test_final_sift/sift_octave1/get_descriptor/scale_space/Gaussian_scale2 ==
  pixel_in : Inport
  valid_in : Inport  Port=2
  Mul : Subsystem
  Round : allblocks_alteradspbuilder2/Round  BusType=Signed Fractional  bwl=9  bwr=16  bitsToRemove=0  roundMode=TRUNCATE_LOW  userRoundMode=Truncate  pipeline=off  pipeline_display=0  use_ena=off  use_aclr=off
  line_buff : Subsystem
  pixel_out : Outport
  wires:
  line_buff/20(Out34) -> Mul/20(In34)
  line_buff/7(Out11) -> Mul/7(In11)
  line_buff/22(Out41) -> Mul/22(In41)
  line_buff/21(Out40) -> Mul/21(In40)
  line_buff/23(Out42) -> Mul/23(In42)
  line_buff/24(Out43) -> Mul/24(In43)
  line_buff/6(Out10) -> Mul/6(In10)
  line_buff/19(Out33) -> Mul/19(In33)
  line_buff/25(Out44) -> Mul/25(In44)
  line_buff/11(Out20) -> Mul/11(In20)
  line_buff/1(Out00) -> Mul/1(In00)
  line_buff/5(Out04) -> Mul/5(In04)
  pixel_in/1 -> line_buff/1(dataIn)
  line_buff/13(Out22) -> Mul/13(In22)
  line_buff/16(Out30) -> Mul/16(In30)
  line_buff/18(Out32) -> Mul/18(In32)
  Mul/1(pixel) -> Round/1
  line_buff/10(Out14) -> Mul/10(In14)
  valid_in/1 -> Mul/26(clken), line_buff/2(clken)
  line_buff/12(Out21) -> Mul/12(In21)
  line_buff/14(Out23) -> Mul/14(In23)
  line_buff/2(Out01) -> Mul/2(In01)
  line_buff/4(Out03) -> Mul/4(In03)
  line_buff/9(Out13) -> Mul/9(In13)
  line_buff/15(Out24) -> Mul/15(In24)
  line_buff/17(Out31) -> Mul/17(In31)
  line_buff/3(Out02) -> Mul/3(In02)
  line_buff/8(Out12) -> Mul/8(In12)
  Round/1 -> pixel_out/1

== system test_final_sift/sift_octave1/get_descriptor/scale_space/Gaussian_scale3 ==
  pixel_in : Inport
  valid_in : Inport  Port=2
  Mul : Subsystem
  Round : allblocks_alteradspbuilder2/Round  BusType=Signed Fractional  bwl=9  bwr=16  bitsToRemove=0  roundMode=TRUNCATE_LOW  userRoundMode=Truncate  pipeline=off  pipeline_display=0  use_ena=off  use_aclr=off
  line_buff : Subsystem
  pixel_out : Outport
  wires:
  line_buff/20(Out34) -> Mul/20(In34)
  line_buff/7(Out11) -> Mul/7(In11)
  line_buff/22(Out41) -> Mul/22(In41)
  line_buff/21(Out40) -> Mul/21(In40)
  line_buff/23(Out42) -> Mul/23(In42)
  line_buff/24(Out43) -> Mul/24(In43)
  line_buff/6(Out10) -> Mul/6(In10)
  line_buff/19(Out33) -> Mul/19(In33)
  line_buff/25(Out44) -> Mul/25(In44)
  line_buff/11(Out20) -> Mul/11(In20)
  line_buff/1(Out00) -> Mul/1(In00)
  line_buff/5(Out04) -> Mul/5(In04)
  pixel_in/1 -> line_buff/1(dataIn)
  line_buff/13(Out22) -> Mul/13(In22)
  line_buff/16(Out30) -> Mul/16(In30)
  line_buff/18(Out32) -> Mul/18(In32)
  Mul/1(pixel) -> Round/1
  line_buff/10(Out14) -> Mul/10(In14)
  valid_in/1 -> Mul/26(clken), line_buff/2(clken)
  line_buff/12(Out21) -> Mul/12(In21)
  line_buff/14(Out23) -> Mul/14(In23)
  line_buff/2(Out01) -> Mul/2(In01)
  line_buff/4(Out03) -> Mul/4(In03)
  line_buff/9(Out13) -> Mul/9(In13)
  line_buff/15(Out24) -> Mul/15(In24)
  line_buff/17(Out31) -> Mul/17(In31)
  line_buff/3(Out02) -> Mul/3(In02)
  line_buff/8(Out12) -> Mul/8(In12)
  Round/1 -> pixel_out/1

== system test_final_sift/sift_octave1/get_descriptor/scale_space/Gaussian_scale4 ==
  pixel_in : Inport
  valid_in : Inport  Port=2
  Mul : Subsystem
  Round : allblocks_alteradspbuilder2/Round  BusType=Signed Fractional  bwl=9  bwr=16  bitsToRemove=0  roundMode=TRUNCATE_LOW  userRoundMode=Truncate  pipeline=off  pipeline_display=0  use_ena=off  use_aclr=off
  line_buff : Subsystem
  pixel_out : Outport
  wires:
  line_buff/20(Out34) -> Mul/20(In34)
  line_buff/7(Out11) -> Mul/7(In11)
  line_buff/22(Out41) -> Mul/22(In41)
  line_buff/21(Out40) -> Mul/21(In40)
  line_buff/23(Out42) -> Mul/23(In42)
  line_buff/24(Out43) -> Mul/24(In43)
  line_buff/6(Out10) -> Mul/6(In10)
  line_buff/19(Out33) -> Mul/19(In33)
  line_buff/25(Out44) -> Mul/25(In44)
  line_buff/11(Out20) -> Mul/11(In20)
  line_buff/1(Out00) -> Mul/1(In00)
  line_buff/5(Out04) -> Mul/5(In04)
  pixel_in/1 -> line_buff/1(dataIn)
  line_buff/13(Out22) -> Mul/13(In22)
  line_buff/16(Out30) -> Mul/16(In30)
  line_buff/18(Out32) -> Mul/18(In32)
  Mul/1(pixel) -> Round/1
  line_buff/10(Out14) -> Mul/10(In14)
  valid_in/1 -> Mul/26(clken), line_buff/2(clken)
  line_buff/12(Out21) -> Mul/12(In21)
  line_buff/14(Out23) -> Mul/14(In23)
  line_buff/2(Out01) -> Mul/2(In01)
  line_buff/4(Out03) -> Mul/4(In03)
  line_buff/9(Out13) -> Mul/9(In13)
  line_buff/15(Out24) -> Mul/15(In24)
  line_buff/17(Out31) -> Mul/17(In31)
  line_buff/3(Out02) -> Mul/3(In02)
  line_buff/8(Out12) -> Mul/8(In12)
  Round/1 -> pixel_out/1
